simulink model "our"  (R2020b)
settings: Solver=FixedStepAuto  StartTime=0.0  StopTime=15  FixedStep=0.001  RelTol=1e-3
values from neighbouring files (symbols this model uses):
  b0 = 20    [energy_aware_setup.m]    (also in our_setup.m = 2 * sqrt(100))
  k0 = 100    [energy_aware_setup.m]    (also in our_setup.m)
  km = 100    [energy_aware_setup.m]    (also in our_setup.m)
  m_R = 1    [energy_aware_setup.m]    (also in our_setup.m)
  t_collision = 0    [energy_aware_setup.m]    (also in our_setup.m)
  x_O = out.clear.Data(:, 1)    [clear_plot.m]    (also in energy_aware.m = out.eaware.Data(:, 1); energy_aware_plot.m = out.eaware.Data(:, 1); energy_aware_setup.m = 0.5; our_plot.m = out.our.Data(:, 1))
  x_R = out.clear.Data(:, 3)    [clear_plot.m]    (also in energy_aware.m = out.eaware.Data(:, 3); energy_aware_plot.m = out.eaware.Data(:, 3); energy_aware_setup.m = 0; our_plot.m = out.our.Data(:, 3))
libraries: simulink x1
settings Model: Creator=kika  LastModifiedBy=kika

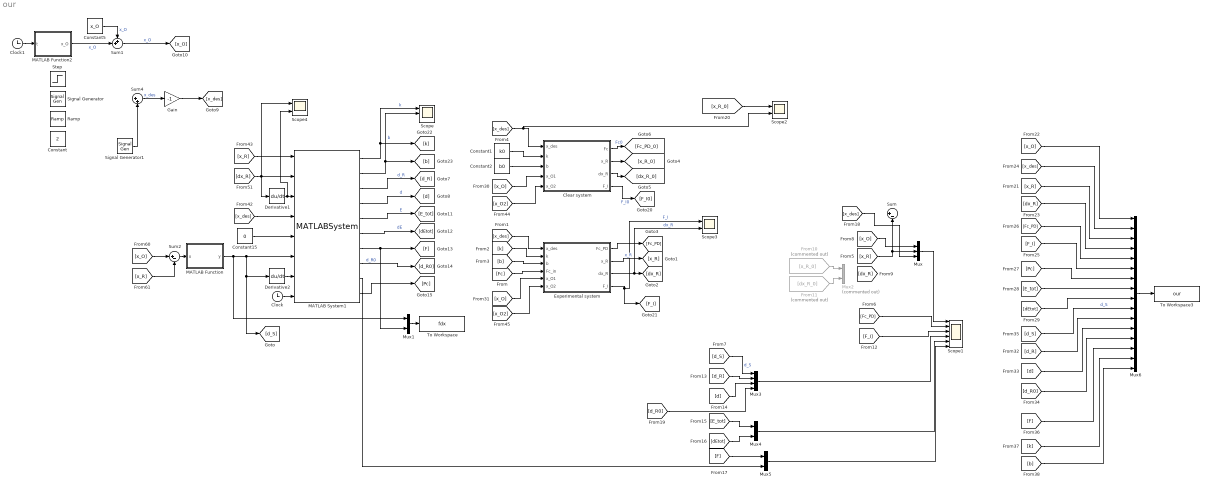
== system our ==
  Clear system : Subsystem
  Clock : Clock
  Clock1 : Clock
  Constant : Constant  Value=2
  Constant1 : Constant  Value=k0
  Constant15 : Constant  Value=0
  Constant2 : Constant  Value=b0
  Constant5 : Constant  Value=x_O
  Derivative1 : Derivative
  Derivative2 : Derivative
  Experimental system : Subsystem
  From10 : From  Commented=on  GotoTag=x_R_0
  From11 : From  Commented=on  GotoTag=dx_R_0
  Gain : Gain  Gain=-1
  MATLAB Function : MATLAB Function  TreatAsAtomicUnit=on
  MATLAB Function2 : MATLAB Function  TreatAsAtomicUnit=on
  MATLAB System1 : MATLABSystem  System=Safety  k0=[k0]  m_R=[1]  j_max=[2000]  F_max=[20]  C_max=[10000]  alpha=[0.01]  SimulateUsing=Code generation
      mask Type: Safety
      mask Display:
      | disp('Safety');
      | port_label('input',1,'x_R');
      | port_label('input',2,'dx_R');
      | port_label('input',3,'ddx_R');
      | port_label('input',4,'x_V');
      | port_label('input',5,'d_O');
      | port_label('input',6,'d_S');
      | port_label('input',7,'dot_d_S');
      | port_label('input',8,'t');
      | port_label('output',1,'k');
      | port_label('output',2,'b');
      | port_label('output',3,'d_R');
      | port_label('output',4,'d');
      | port_label('output',5,'E');
      | port_label('output',6,'dE');
      | port_label('output',7,'F');
      | port_label('output',8,'d_R0');
      | port_label('output',9,'F_star');
      | port_label('output',10,'Pc');
  Mux : Mux  Inputs=3
  Mux1 : Mux  Inputs=2
  Mux2 : Mux  Commented=on  Inputs=2
  Mux3 : Mux
  Mux4 : Mux  Inputs=2
  Mux5 : Mux  Inputs=2
  Mux6 : Mux  Inputs=16
  Ramp : simulink/Sources/Ramp  slope=1  start=0  InitialOutput=0
  Scope : Scope  NumInputPorts=3
  Scope1 : Scope  NumInputPorts=6
  Scope2 : Scope  NumInputPorts=2
  Scope3 : Scope  NumInputPorts=2
  Scope4 : Scope  NumInputPorts=2
  Signal Generator : SignalGenerator  Frequency=0.5  Units=rad/sec
  Signal Generator1 : SignalGenerator  Amplitude=4  Units=rad/sec
  Step : Step  Time=10  Before=1  After=0  SampleTime=0
  Sum : Sum  Inputs=|+-
  Sum1 : Sum  Inputs=++|
  Sum2 : Sum  Inputs=|+-
  Sum4 : Sum  Inputs=|++
  To Workspace : ToWorkspace  VariableName=fdx  SaveFormat=Timeseries  SampleTime=-1
  To Workspace3 : ToWorkspace  VariableName=our  SaveFormat=Timeseries  SampleTime=-1
  wires:
  [Fc] -> Experimental system/4(Fc_in)
  [x_des] -> Experimental system/1(x_des)
  Experimental system/2(x_R) -> [x_R]  "x_R"
  Experimental system/3(dx_R) -> Scope3/2, [dx_R]  "dx_R"
  Experimental system/1(Fc_PD) -> [Fc_PD]
  Clear system/1(Fc) -> [Fc_PD_0]  "Fc0"
  Clear system/2(x_R) -> [x_R_0]
  Clear system/3(dx_R) -> [dx_R_0]
  [k] -> Experimental system/2(k)
  [b] -> Experimental system/3(b)
  [x_des] -> Scope2/2, Clear system/1(x_des)
  Constant1/1 -> Clear system/2(k)
  Constant2/1 -> Clear system/3(b)
  Sum4/1 -> Gain/1  "x_des"
  [x_O] -> Experimental system/5(x_O1)
  [x_O] -> Clear system/4(x_O1)
  Constant5/1 -> Sum1/1  "x_O"
  Sum1/1 -> [x_O]  "x_O"
  MATLAB Function2/1(x_O) -> Sum1/2  "x_O"
  Clock1/1 -> MATLAB Function2/1(t)
  Clear system/4(F_I) -> [F_I0]  "F_I0"
  Experimental system/4(F_I) -> [F_I], Scope3/1  "F_I"
  [x_O2] -> Clear system/5(x_O2)
  [x_O2] -> Experimental system/6(x_O2)
  Constant15/1 -> MATLAB System1/5
  [x_des] -> MATLAB System1/4
  [x_R] -> MATLAB System1/1
  [dx_R] -> Scope4/1, Derivative1/1, MATLAB System1/2
  Derivative2/1 -> MATLAB System1/7
  Sum2/1 -> MATLAB Function/1(u)
  [x_O] -> Sum2/1
  [x_R] -> Sum2/2
  MATLAB System1/1 -> Scope/1, [k]  "k"
  Derivative1/1 -> Scope4/2, MATLAB System1/3
  MATLAB System1/2 -> [b], Scope/2  "b"
  [x_R] -> Sum/2, Mux/2
  [Fc_PD] -> Scope1/2
  MATLAB System1/4 -> [d]  "d"
  Mux/1 -> Scope1/1
  [x_O] -> Mux/1
  MATLAB Function/1(y) -> MATLAB System1/6, [d_S], Derivative2/1, Mux1/1
  MATLAB System1/7 -> Mux1/2, [F]
  Clock/1 -> MATLAB System1/8
  Mux1/1 -> To Workspace/1
  From10/1 -> Mux2/1
  From11/1 -> Mux2/2
  [F_I] -> Scope1/3
  MATLAB System1/3 -> [d_R]  "d_R"
  MATLAB System1/5 -> [E_tot]  "E"
  MATLAB System1/6 -> [dEtot]  "dE"
  [d_R] -> Mux3/2
  [d_S] -> Mux3/1  "d_S"
  [d] -> Mux3/3
  [E_tot] -> Mux4/1
  [dEtot] -> Mux4/2
  Mux3/1 -> Scope1/4
  Mux4/1 -> Scope1/5
  [F] -> Mux5/1
  [x_des] -> Mux/3
  MATLAB System1/8 -> [d_R0]  "d_R0"
  [d_R0] -> Mux3/4
  Mux5/1 -> Scope1/6
  MATLAB System1/9 -> Mux5/2
  Signal Generator1/1 -> Sum4/2
  [x_R_0] -> Scope2/1
  Gain/1 -> [x_des]
  MATLAB System1/10 -> [Pc]
  [dx_R] -> Mux6/4
  [x_R] -> Mux6/3
  [Fc_PD] -> Mux6/5
  [x_des] -> Mux6/2
  [F_I] -> Mux6/6
  [x_O] -> Mux6/1
  [Pc] -> Mux6/7
  [E_tot] -> Mux6/8
  [dEtot] -> Mux6/9
  [d_S] -> Mux6/10  "d_S"
  [d_R] -> Mux6/11
  [d] -> Mux6/12
  [d_R0] -> Mux6/13
  [F] -> Mux6/14
  [k] -> Mux6/15
  [b] -> Mux6/16
  Mux6/1 -> To Workspace3/1

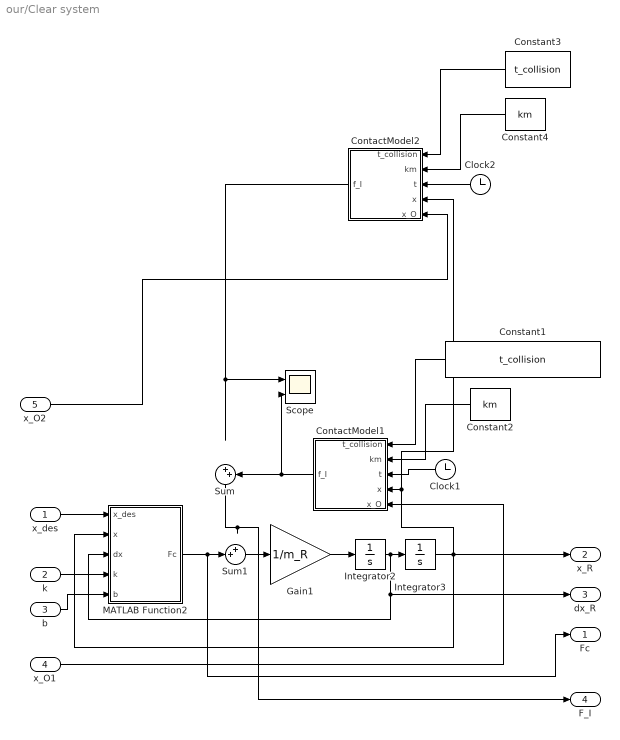
== system our/Clear system ==
  x_des : Inport
  k : Inport  Port=2
  b : Inport  Port=3
  x_O1 : Inport  Port=4
  x_O2 : Inport  Port=5
  Clock1 : Clock
  Clock2 : Clock
  Constant1 : Constant  Value=t_collision
  Constant2 : Constant  Value=km
  Constant3 : Constant  Value=t_collision
  Constant4 : Constant  Value=km
  ContactModel1 : MATLAB Function  TreatAsAtomicUnit=on
  ContactModel2 : MATLAB Function  TreatAsAtomicUnit=on
  Gain1 : Gain  Gain=1/m_R
  Integrator2 : Integrator
  Integrator3 : Integrator  InitialCondition=x_R
  MATLAB Function2 : MATLAB Function  TreatAsAtomicUnit=on
  Scope : Scope  NumInputPorts=2
  Sum : Sum  Inputs=|++
  Sum1 : Sum  Inputs=++|
  Fc : Outport
  x_R : Outport  Port=2
  dx_R : Outport  Port=3
  F_I : Outport  Port=4
  wires:
  k/1 -> MATLAB Function2/4(k)
  ContactModel1/1(f_I) -> Sum/2, Scope/2
  Clock1/1 -> ContactModel1/3(t)
  x_des/1 -> MATLAB Function2/1(x_des)
  b/1 -> MATLAB Function2/5(b)
  Sum1/1 -> Gain1/1
  x_O1/1 -> ContactModel1/5(x_O)
  Gain1/1 -> Integrator2/1
  MATLAB Function2/1(Fc) -> Fc/1, Sum1/2
  Integrator2/1 -> dx_R/1, MATLAB Function2/3(dx), Integrator3/1
  Constant1/1 -> ContactModel1/1(t_collision)
  Constant2/1 -> ContactModel1/2(km)
  Constant3/1 -> ContactModel2/1(t_collision)
  Integrator3/1 -> x_R/1, ContactModel2/4(x), ContactModel1/4(x), MATLAB Function2/2(x)
  x_O2/1 -> ContactModel2/5(x_O)
  Constant4/1 -> ContactModel2/2(km)
  Clock2/1 -> ContactModel2/3(t)
  Sum/1 -> F_I/1
  ContactModel2/1(f_I) -> Scope/1

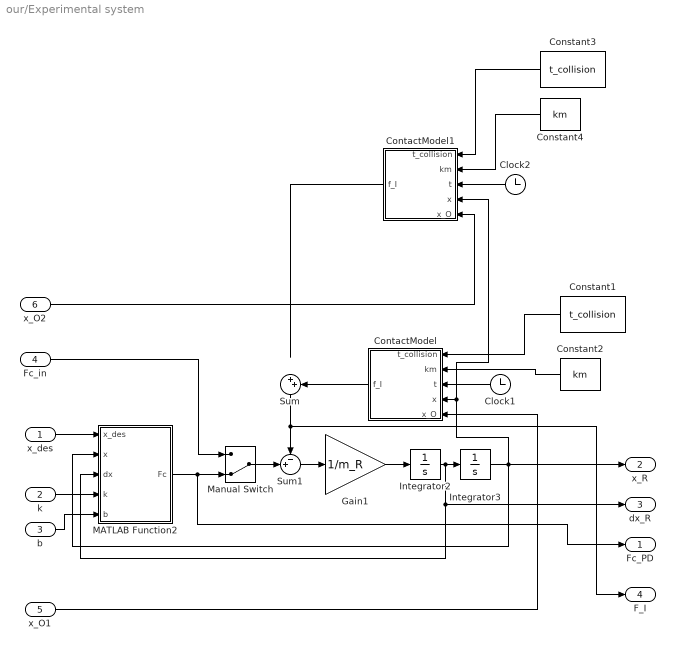
== system our/Experimental system ==
  x_des : Inport
  k : Inport  Port=2
  b : Inport  Port=3
  Fc_in : Inport  Port=4
  x_O1 : Inport  Port=5
  x_O2 : Inport  Port=6
  Clock1 : Clock
  Clock2 : Clock
  Constant1 : Constant  Value=t_collision
  Constant2 : Constant  Value=km
  Constant3 : Constant  Value=t_collision
  Constant4 : Constant  Value=km
  ContactModel : MATLAB Function  TreatAsAtomicUnit=on
  ContactModel1 : MATLAB Function  TreatAsAtomicUnit=on
  Gain1 : Gain  Gain=1/m_R
  Integrator2 : Integrator
  Integrator3 : Integrator  InitialCondition=x_R
  MATLAB Function2 : MATLAB Function  TreatAsAtomicUnit=on
  Manual Switch : ManualSwitch  CurrentSetting=0
  Sum : Sum  Inputs=|++
  Sum1 : Sum  Inputs=-+|
  Fc_PD : Outport
  x_R : Outport  Port=2
  dx_R : Outport  Port=3
  F_I : Outport  Port=4
  wires:
  k/1 -> MATLAB Function2/4(k)
  ContactModel/1(f_I) -> Sum/2
  Clock1/1 -> ContactModel/3(t)
  Integrator3/1 -> x_R/1, ContactModel1/4(x), ContactModel/4(x), MATLAB Function2/2(x)
  x_des/1 -> MATLAB Function2/1(x_des)
  b/1 -> MATLAB Function2/5(b)
  Sum1/1 -> Gain1/1
  x_O1/1 -> ContactModel/5(x_O)
  Gain1/1 -> Integrator2/1
  MATLAB Function2/1(Fc) -> Manual Switch/2, Fc_PD/1
  Integrator2/1 -> dx_R/1, MATLAB Function2/3(dx), Integrator3/1
  Constant1/1 -> ContactModel/1(t_collision)
  Constant2/1 -> ContactModel/2(km)
  Fc_in/1 -> Manual Switch/1
  Manual Switch/1 -> Sum1/2
  ContactModel1/1(f_I) -> ?
  Constant4/1 -> ContactModel1/2(km)
  Constant3/1 -> ContactModel1/1(t_collision)
  Clock2/1 -> ContactModel1/3(t)
  x_O2/1 -> ContactModel1/5(x_O)
  Sum/1 -> F_I/1, Sum1/1

== matlab function our/Experimental system/ContactModel ==
  data: t_collision input; km input; t input; f_I output; x input; x_O input
function f_I = fcn(t_collision, km, t, x, x_O)


f_I = 0;

if t > t_collision
    if x > x_O
        f_I = km * (x - x_O);
    end
end

% if t > t_collision
%     if abs(x) - abs(x_O) > 0
%         f_I = km * (abs(x_O) - abs(x));
%     end
% end

== matlab function our/Experimental system/MATLAB Function2 ==
  data: x_des input; Fc output; x input; dx input; k input; b input
function Fc = fcn(x_des, x, dx, k, b)

Fc = k * (x_des - x) - b * dx;

== matlab function our/MATLAB Function ==
  data: u input; y output
function y = fcn(u)
    
    y = u;

    if u <= 0
        y = 0;
    end

== matlab function our/Clear system/MATLAB Function2 ==
  data: x_des input; Fc output; x input; dx input; k input; b input
function Fc = fcn(x_des, x, dx, k, b)

Fc = k * (x_des - x) - b * dx;

== matlab function our/Clear system/ContactModel1 ==
  data: t_collision input; km input; t input; f_I output; x input; x_O input
function f_I = fcn(t_collision, km, t, x, x_O)


f_I = 0;

if t > t_collision
    if x > x_O
        f_I = km * (x_O - x);    
    end
end

% if t > t_collision
%     if abs(x) - abs(x_O) > 0
%         f_I = km * (abs(x_O) - abs(x));
%     end
% end

== matlab function our/MATLAB Function2 ==
  data: t input; x_O output
function x_O = fcn(t)

    x_O = 3.5;
    if t > 8
        x_O = 0;
    end
%         
%     offset = -0.3;
%     x_O = 1;
%     if t > 23 && t < 35
%         x_O = sin(0.5 * t + pi);
%     end
%     if t >= offset + 44.5 && t < offset +46.8
%         x_O = 2*sin(1.5 * t - pi/6);
%     end
%     if t > 85
%         x_O = 0.2;
%     end
%

== matlab function our/Experimental system/ContactModel1 ==
  data: t_collision input; km input; t input; f_I output; x input; x_O input
function f_I = fcn(t_collision, km, t, x, x_O)


f_I = 0;

if t > t_collision
    if x < x_O
        f_I = km * (x - x_O);
    end
end

== matlab function our/Clear system/ContactModel2 ==
  data: t_collision input; km input; t input; f_I output; x input; x_O input
function f_I = fcn(t_collision, km, t, x, x_O)


f_I = 0;


if t > t_collision
    if x < x_O
        f_I = km * (x_O - x);
    end
end
